simulink model "absmdl_Comparison"  (R2023a)
settings: Solver=ode45  StartTime=0  StopTime=15  FixedStep=0.002  RelTol=1e-3  AbsTol=1e-6
libraries: Solver_SF x1
settings Model: ExtModeTrigMode=oneshot  Creator=pmather  LastModifiedBy=USER
settings SolverCC: AutoScaleAbsTol=off  AlgebraicLoopSolver=TrustRegion
settings DataIOCC: SaveFormat=Array  SignalLoggingSaveFormat=ModelDataLogs  ReturnWorkspaceOutputs=off
settings OptimizationCC: BlockReduction=off  BooleanDataType=off  ExpressionDepthLimit=2147483647  InitFltsAndDblsToZero=on  LifeSpan=inf
settings DebuggingCC: SaveWithParameterizedLinksMsg=none  UnderspecifiedInitializationDetection=Classic  MergeDetectMultiDrivingBlocksExec=none  SignalResolutionControl=TryResolveAllWithWarning  MultiTaskDSMMsg=warning  MultiTaskCondExecSysMsg=none  FcnCallInpInsideContextMsg=warning  UnconnectedInputMsg=warning  UnconnectedOutputMsg=warning  UnconnectedLineMsg=warning  StateNameClashWarn=warning  SFUnexpectedBacktrackingDiag=warning  SFNoUnconditionalDefaultTransitionDiag=warning  SFExecutionAtInitializationDiag=none  ArithmeticOperatorsInVariantConditions=warning
settings HardwareCC: ProdBitPerPointer=32  ProdBitPerSizeT=32  ProdBitPerPtrDiffT=32  ProdLargestAtomicFloat=None  ProdIntDivRoundTo=Undefined  ProdEndianess=Unspecified  ProdWordSize=32  ProdHWDeviceType=32-bit Generic  TargetUnknown=on
settings ModelReferenceCC: PropagateSignalLabelsOutOfModel=off
settings SFSimCC: SimUseLocalCustomCode=off  CustomCodeUndefinedFunction=UseInterfaceOnly
settings RTWCC: TemplateMakefile=grt_vc.tmf  RTWUseLocalCustomCode=off
settings CodeAppCC: StateflowObjectComments=on
settings GRTTargetCC: TargetLangStandard=C89/C90 (ANSI)  CombineOutputUpdateFcns=off  GRTInterface=on
settings ConfigComp: CovMetricSettings=dw  CovSaveCumulativeToWorkspaceVar=on  CovSaveSingleToWorkspaceVar=on  CovExternalEMLEnable=off

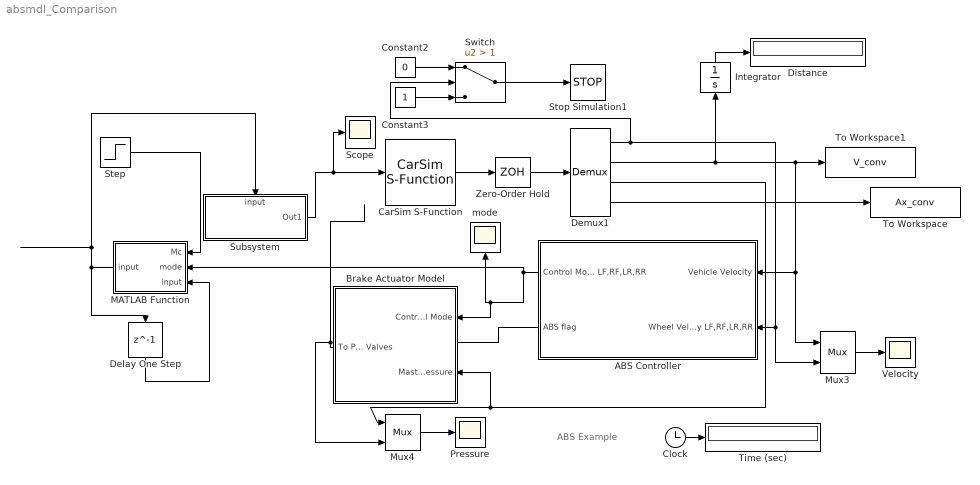
== system absmdl_Comparison ==
  note: ABS Example
  ABS Controller : Subsystem
  Brake Actuator Model : Subsystem
  CarSim S-Function : Solver_SF/CarSim S-Function  Priority=1  SIMFILE=simfile.sim  Run_RTs=off  vs_state_ind=Run  StopMode_ind=Vehicle Model
  Clock : Clock
  Constant2 : Constant  Value=0
  Constant3 : Constant
  Delay One Step : Delay  DelayLength=1  InitialCondition=[0 0 0 0]'  SampleTime=0.01
  Demux1 : Demux  Outputs=[4 1 1 1]
      settings: DisplayOption=none
  Distance : Display
      settings: Format=bank  Decimation=100
  Integrator : Integrator
  MATLAB Function : MATLAB Function  TreatAsAtomicUnit=on
  Mux3 : Mux  Inputs=2
  Mux4 : Mux  Inputs=2
  Pressure : Scope
  Scope : Scope
  Step : Step  Time=5  After=5  SampleTime=0.01
  Stop Simulation1 : Stop
  Subsystem : Subsystem
      settings: PortSchema="{\"entries\":[{\"content\":{\"sides\":[{\"content\":{},\"type\":\"ConnectorPlacement.EquallySpacedRectSide\",\"uuid\":\"4213256a-b74f-4c4a-9dc0-d014229249a7\"},{\"content\":{\"connectorIds\":[\"Out1\"],\"side\":\"RIGHT\"},\"type\":\"ConnectorPlacement.EquallySpacedRectSide\",\"uuid\":\"31df4868-331a-4411-820f-93eb39f46ca6\"},{\"content\":{\"connectorIds\":[\"In1\"],\"side\":\"TOP\"},\"type\":\"ConnectorPlacement.EquallySpacedRectSide\",\"uuid\":\"471b8cdd-c059-4f79-bfb9-76dd5bcdb307\"}]},\"type\":\"ConnectorPlacement.EquallySpacedConnector\",\"uuid\":\"f67c12da-0db3-482f-ad54-3a65f26df550\"}],\"packageUris\":[\"http://schema.mathworks.com/mf0/Connector/R2020b\"],\"version\":\"1.0\"}"
  Switch : Switch  Criteria=u2 > Threshold  Threshold=1  SaturateOnIntegerOverflow=off  InputSameDT=off
  Time (sec) : Display
      settings: Format=bank  Decimation=100
  To Workspace : ToWorkspace  VariableName=Ax_conv  SaveFormat=Timeseries  SampleTime=-1
  To Workspace1 : ToWorkspace  VariableName=V_conv  SaveFormat=Timeseries  SampleTime=-1
  Velocity : Scope
  Zero-Order Hold : ZeroOrderHold  SampleTime=0.01
  mode : Scope
  wires:
  Mux4/1 -> Pressure/1
  CarSim S-Function/1 -> Zero-Order Hold/1
  Demux1/2 -> To Workspace1/1, Mux3/1, ABS Controller/1(Vehicle Velocity), Integrator/1
  Clock/1 -> Time (sec)/1
  ABS Controller/1(Control Mode LF,RF,LR,RR) -> mode/1, Brake Actuator Model/1(Control Mode), MATLAB Function/2(mode)
  Brake Actuator Model/1(To Propotional Valves) -> Mux4/2
  Mux3/1 -> Velocity/1
  Demux1/3 -> Mux4/1, Brake Actuator Model/2(Master Pressure)
  ABS Controller/2(ABS flag) -> ?
  Step/1 -> MATLAB Function/1(Mc)
  MATLAB Function/1(input) -> Subsystem/1(input), Delay One Step/1
  Delay One Step/1 -> MATLAB Function/3("input ")
  Zero-Order Hold/1 -> Demux1/1
  Subsystem/1(Out1) -> CarSim S-Function/1, Scope/1
  Constant2/1 -> Switch/1
  Demux1/1 -> Switch/2, Mux3/2, ABS Controller/2(Wheel Velocity LF,RF,LR,RR)
  Switch/1 -> Stop Simulation1/1
  Constant3/1 -> Switch/3
  Demux1/4 -> To Workspace/1
  Integrator/1 -> Distance/1

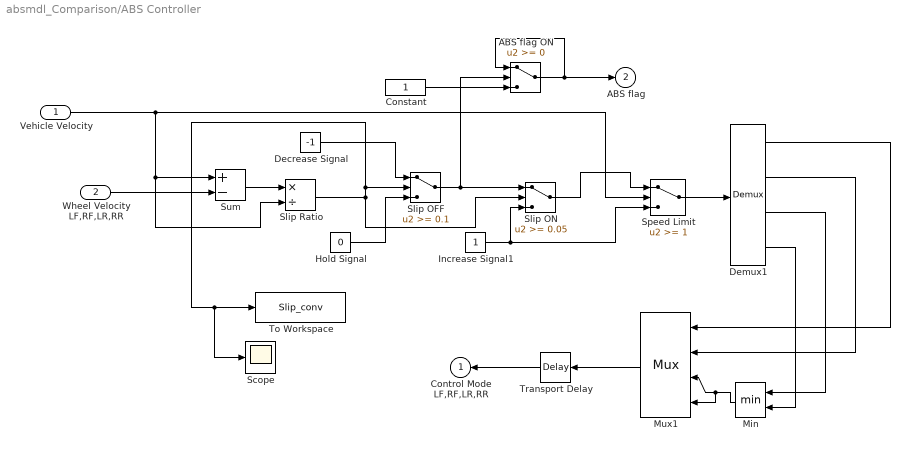
== system absmdl_Comparison/ABS Controller ==
  Vehicle Velocity : Inport
  Wheel Velocity LF,RF,LR,RR : Inport  Port=2
  ABS flag ON : Switch
  Constant : Constant
  Decrease Signal : Constant  Value=-1
  Demux1 : Demux
      settings: DisplayOption=none
  Hold Signal : Constant  Value=0
  Increase Signal1 : Constant
  Min : MinMax  Inputs=2  InputSameDT=on  SaturateOnIntegerOverflow=on
  Mux1 : Mux
  Scope : Scope
  Slip OFF : Switch  Threshold=0.1
  Slip ON : Switch  Threshold=0.05
  Slip Ratio : Product  Inputs=*/  InputSameDT=on  RndMeth=Zero  SaturateOnIntegerOverflow=on  OutDataTypeStr=Inherit: Same as first input
  Speed Limit : Switch  Threshold=1
  Sum : Sum  Inputs=+-  InputSameDT=on  SaturateOnIntegerOverflow=on  OutDataTypeStr=Inherit: Same as first input
  To Workspace : ToWorkspace  VariableName=Slip_conv  SaveFormat=Timeseries  SampleTime=-1
  Transport Delay : TransportDelay  DelayTime=0.005
  Control Mode LF,RF,LR,RR : Outport  InitialOutput=0
  ABS flag : Outport  Port=2  InitialOutput=0
  wires:
  Decrease Signal/1 -> Slip OFF/1
  Sum/1 -> Slip Ratio/1
  Wheel Velocity LF,RF,LR,RR/1 -> Sum/2
  Slip OFF/1 -> ABS flag ON/2, Slip ON/1
  Vehicle Velocity/1 -> Sum/1, Slip Ratio/2, Speed Limit/2
  Slip ON/1 -> Speed Limit/1
  Increase Signal1/1 -> Slip ON/3, Speed Limit/3
  Slip Ratio/1 -> Scope/1, To Workspace/1, Slip OFF/2, Slip ON/2
  Hold Signal/1 -> Slip OFF/3
  Transport Delay/1 -> Control Mode LF,RF,LR,RR/1
  Speed Limit/1 -> Demux1/1
  Min/1 -> Mux1/3, Mux1/4
  Demux1/2 -> Mux1/2
  Demux1/1 -> Mux1/1
  Mux1/1 -> Transport Delay/1
  Demux1/4 -> Min/2
  Demux1/3 -> Min/1
  Constant/1 -> ABS flag ON/3
  ABS flag ON/1 -> ABS flag/1, ABS flag ON/1

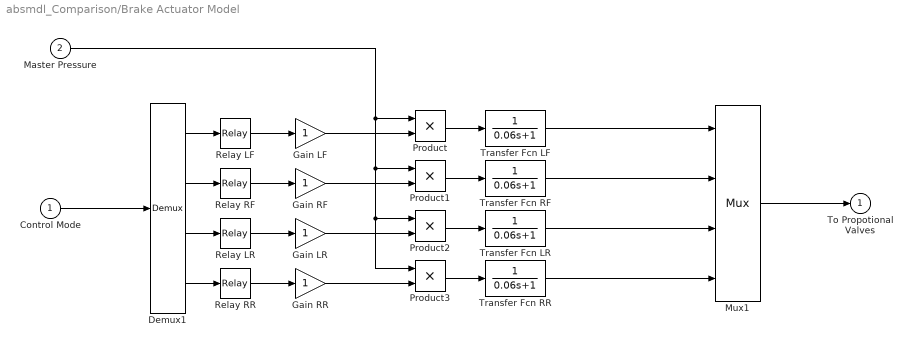
== system absmdl_Comparison/Brake Actuator Model ==
  Control Mode : Inport
  Master Pressure : Inport  Port=2
  Demux1 : Demux
      settings: DisplayOption=none
  Gain LF : Gain  SaturateOnIntegerOverflow=on  OutDataTypeStr=Inherit: Same as input  ParamDataTypeStr=Inherit: Same as input
  Gain LR : Gain  SaturateOnIntegerOverflow=on  OutDataTypeStr=Inherit: Same as input  ParamDataTypeStr=Inherit: Same as input
  Gain RF : Gain  SaturateOnIntegerOverflow=on  OutDataTypeStr=Inherit: Same as input  ParamDataTypeStr=Inherit: Same as input
  Gain RR : Gain  SaturateOnIntegerOverflow=on  OutDataTypeStr=Inherit: Same as input  ParamDataTypeStr=Inherit: Same as input
  Mux1 : Mux
  Product{,1..3} (4 alike) : Product  InputSameDT=on  RndMeth=Zero  SaturateOnIntegerOverflow=on  OutDataTypeStr=Inherit: Same as first input
  Relay LF : Relay  OnSwitchValue=0.5  OffSwitchValue=-0.5
  Relay LR : Relay  OnSwitchValue=0.5  OffSwitchValue=-0.5
  Relay RF : Relay  OnSwitchValue=0.5  OffSwitchValue=-0.5
  Relay RR : Relay  OnSwitchValue=0.5  OffSwitchValue=-0.5
  Transfer Fcn LF : TransferFcn  Denominator=[0.06 1]
  Transfer Fcn LR : TransferFcn  Denominator=[0.06 1]
  Transfer Fcn RF : TransferFcn  Denominator=[0.06 1]
  Transfer Fcn RR : TransferFcn  Denominator=[0.06 1]
  To Propotional Valves : Outport  InitialOutput=0
  wires:
  Mux1/1 -> To Propotional Valves/1
  Control Mode/1 -> Demux1/1
  Demux1/1 -> Relay LF/1
  Demux1/2 -> Relay RF/1
  Demux1/3 -> Relay LR/1
  Demux1/4 -> Relay RR/1
  Relay LF/1 -> Gain LF/1
  Relay RF/1 -> Gain RF/1
  Relay LR/1 -> Gain LR/1
  Relay RR/1 -> Gain RR/1
  Gain LF/1 -> Product/2
  Gain RF/1 -> Product1/2
  Gain LR/1 -> Product2/2
  Gain RR/1 -> Product3/2
  Product/1 -> Transfer Fcn LF/1
  Product1/1 -> Transfer Fcn RF/1
  Product2/1 -> Transfer Fcn LR/1
  Product3/1 -> Transfer Fcn RR/1
  Transfer Fcn RF/1 -> Mux1/2
  Transfer Fcn LR/1 -> Mux1/3
  Transfer Fcn RR/1 -> Mux1/4
  Master Pressure/1 -> Product/1, Product1/1, Product2/1, Product3/1
  Transfer Fcn LF/1 -> Mux1/1

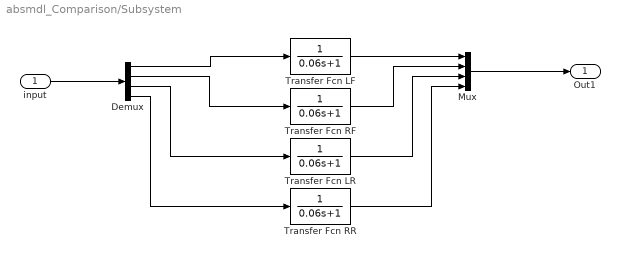
== system absmdl_Comparison/Subsystem ==
  input : Inport
  Demux : Demux
  Mux : Mux
  Transfer Fcn LF : TransferFcn  Denominator=[0.06 1]
  Transfer Fcn LR : TransferFcn  Denominator=[0.06 1]
  Transfer Fcn RF : TransferFcn  Denominator=[0.06 1]
  Transfer Fcn RR : TransferFcn  Denominator=[0.06 1]
  Out1 : Outport
  wires:
  input/1 -> Demux/1
  Demux/1 -> Transfer Fcn LF/1
  Demux/2 -> Transfer Fcn RF/1
  Demux/3 -> Transfer Fcn LR/1
  Demux/4 -> Transfer Fcn RR/1
  Transfer Fcn LF/1 -> Mux/1
  Transfer Fcn RF/1 -> Mux/2
  Transfer Fcn LR/1 -> Mux/3
  Transfer Fcn RR/1 -> Mux/4
  Mux/1 -> Out1/1

== matlab function absmdl_Comparison/MATLAB Function ==
  data: Mc input; mode input; input output; input input
function input = fcn(Mc, mode, input)

if mode(1) == -1
    input(1) = 1;
elseif mode(1) == 0
    input(1) = input(1);%+Mc*0.01;
else
    input(1) = input(1)+Mc/0.3*0.01;
end
if mode(2) == -1
    input(2) = 1;
elseif mode(2) == 0
    input(2) = input(2);%+Mc*0.01;
else
    input(2) = input(2)+Mc/0.3*0.01;
end
if mode(3) == -1
    input(3) = 1;
elseif mode(3) == 0
    input(3) = input(3);%+Mc*0.01;
else
    input(3) = input(3)+Mc/0.3*0.01;
end
if mode(4) == -1
    input(4) = 1;
elseif mode(4) == 0
    input(4) = input(4);%+Mc*0.01;
else
    input(4) = input(4)+Mc/0.3*0.01;
end
